simulink model "a211"  (R2016a)
settings: Solver=VariableStepAuto  StartTime=0.0  StopTime=10.0  RelTol=1e-3
libraries: simCryogenics_lib x5, nesl_utility x4, fl_lib x1
settings Model: Creator=FB229602  LastModifiedBy=FB229602

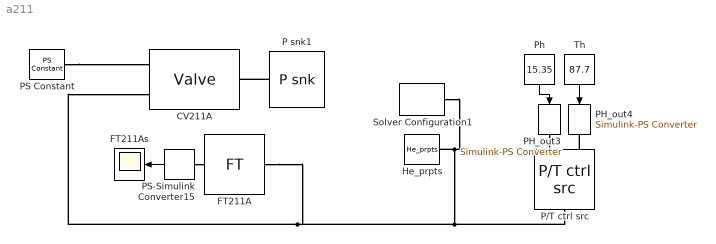
== system a211 ==
  CV211A : simCryogenics_lib/Elements/Valve  CVmax=186  ControlInputMin=0  ControlInputMax=100  Xt=0.86  Rv=50  lin_v=0  lim_v=0  K=2.4e-5 m^1.50000*kg^0.50000/s/bar^0.50000  Cmd_specify=off  Cmd_priority=None  Cmd=0  gamma_specify=off  gamma_priority=None  gamma=0  rho_specify=off  rho_priority=None  rho=0 kg/m^3  Xc_specify=off  Xc_priority=None  Xc=0  X_specify=off  X_priority=None  X=0  Y_specify=off  Y_priority=None  Y=0  CV_specify=off  CV_priority=None  CV=0
  FT211A : simCryogenics_lib/Sensors/FT
  FT211As : Scope
  He_prpts : simCryogenics_lib/Utilities/He_prpts  P_min=0.25 bar  P_max=20 bar  T_min=3 K  T_max=320 K  N=100  Mol=4.0026 * 10 ^ (- 3) kg/mol
  P snk1 : simCryogenics_lib/Sources_Sinks/P snk  P=15.28 bar
  P/T ctrl src : simCryogenics_lib/Sources_Sinks/P//T ctrl src
  PH_out3 : nesl_utility/Simulink-PS Converter  PhysicalDomain=network_engine_domain  SubClassName=ps_input  LeftPortType=input  RightPortType=output  PseudoPeriodic=off  Frequencies=[]  NoiseDistribution=none  NoiseParameters=[]  Unit=bar  AffineConversion=off  InputFiltering=off  SimscapeFilterOrder=1  InputFilterTimeConstant=0.001  UdotUserProvided=1
  PH_out4 : nesl_utility/Simulink-PS Converter  PhysicalDomain=network_engine_domain  SubClassName=ps_input  LeftPortType=input  RightPortType=output  PseudoPeriodic=off  Frequencies=[]  NoiseDistribution=none  NoiseParameters=[]  Unit=K  AffineConversion=off  InputFiltering=off  SimscapeFilterOrder=1  InputFilterTimeConstant=0.001  UdotUserProvided=1
  PS Constant : fl_lib/Physical Signals/Sources/PS Constant  constant=O
  PS-Simulink Converter15 : nesl_utility/PS-Simulink Converter  PhysicalDomain=network_engine_domain  SubClassName=ps_output  LeftPortType=input  RightPortType=output  PseudoPeriodic=off  Frequencies=[]  Unit=1  AffineConversion=off
  Ph : Constant  Value=15.35
  Solver Configuration1 : nesl_utility/Solver Configuration  PhysicalDomain=network_engine_domain  SubClassName=solver  LeftPortType=input  RightPortType=generic  Accelerate=off  Tones=[]  Harmonics=[]  SimulateNoise=off  Profile=off  UseLocalSampling=off  EnableSwitchedLinearOptims=on  FrequencyDomain=off  UseCCode=off  RelTol=0.001  AbsTol=1e-06  MinStep=1e-09  ToWorkspace=off  RevertToSquareIcSolve=off  NumHomotopyIterations=100  PhasorMode=off  PhasorModeNumHarmonics=1  OverrideAbsTol=off  DoDC=off  ResidualTolerance=1e-09  UseLocalSolver=off  LocalSolverChoice=NE_BACKWARD_EULER_ADVANCER  LocalSolverSampleTime=20  DoFixedCost=off  MaxNonlinIter=10  MaxModeIter=2  LinearAlgebra=Sparse  DelaysMemoryBudget=1024  AutomaticFiltering=on  FilteringTimeConstant=0.001
  Th : Constant  Value=87.7
  wires:
  Th/1 -> PH_out4/1
  Ph/1 -> PH_out3/1
  PS-Simulink Converter15/1 -> FT211As/1
  connections:
  P snk1/RConn1 -- CV211A/RConn1
  PS Constant/RConn1 -- CV211A/LConn1
  P/T ctrl src/LConn2 -- PH_out4/RConn1
  PH_out3/RConn1 -- P/T ctrl src/LConn1
  He_prpts/RConn1 -- Solver Configuration1/RConn1 -- FT211A/LConn1 -- CV211A/LConn2 -- P/T ctrl src/RConn1
  PS-Simulink Converter15/LConn1 -- FT211A/RConn1
